simulink model "SimulationLab2"  (R2020a)
settings: Solver=VariableStepAuto  StartTime=0.0  StopTime=20  MaxStep=0.001  RelTol=1e-3
model workspace (MAT data in the model file):
  Phi21 = Simulink.Parameter
  Phi21.DataType = 'auto'
  Phi21.Dimensions = [0 0]
values from neighbouring files (symbols this model uses):
  b = 0.3    [SimLab2_MATLAB.m]
  d0 = 0    [SimLab2_MATLAB.m]
  ddot0 = 0    [SimLab2_MATLAB.m]
  Gamma1 = Gamma(end)    [SimLab2_MATLAB.m]
  Gamma2 = Gamma(1:end-1)    [SimLab2_MATLAB.m]
  H = [0 0 0 1]    [SimLab2_MATLAB.m]
  k = 32    [SimLab2_MATLAB.m]
  K = place(Phi,Gamma,P)    [SimLab2_MATLAB.m]
  L = place(Phi',H',Po)'    [SimLab2_MATLAB.m]
  Lr = place(Phi22',Phi12',Pr)'    [SimLab2_MATLAB.m]
  M = 20    [SimLab2_MATLAB.m]
  m = 1    [SimLab2_MATLAB.m]
  N = Nu + K*Nx    [SimLab2_MATLAB.m]
  noise = 0    [SimLab2_MATLAB.m]
  Phi11 = Phi(end,end)    [SimLab2_MATLAB.m]
  Phi12 = Phi(end,1:end-1)    [SimLab2_MATLAB.m]
  Phi21 = Phi(1:end-1,end)    [SimLab2_MATLAB.m]
  Phi22 = Phi(1:end-1,1:end-1)    [SimLab2_MATLAB.m]
  sat = 10    [SimLab2_MATLAB.m]
  T = 1/f    (= 0.2)    [SimLab2_MATLAB.m]
  xhat0 = 0    [SimLab2_MATLAB.m]
  y0 = 0    [SimLab2_MATLAB.m]
  ydot0 = 0    [SimLab2_MATLAB.m]
undefined symbols (not defined in the file or in its folder): Gamma, Phi
libraries: dspsrcs4 x2
settings Model: Creator=moham  LastModifiedBy=moham

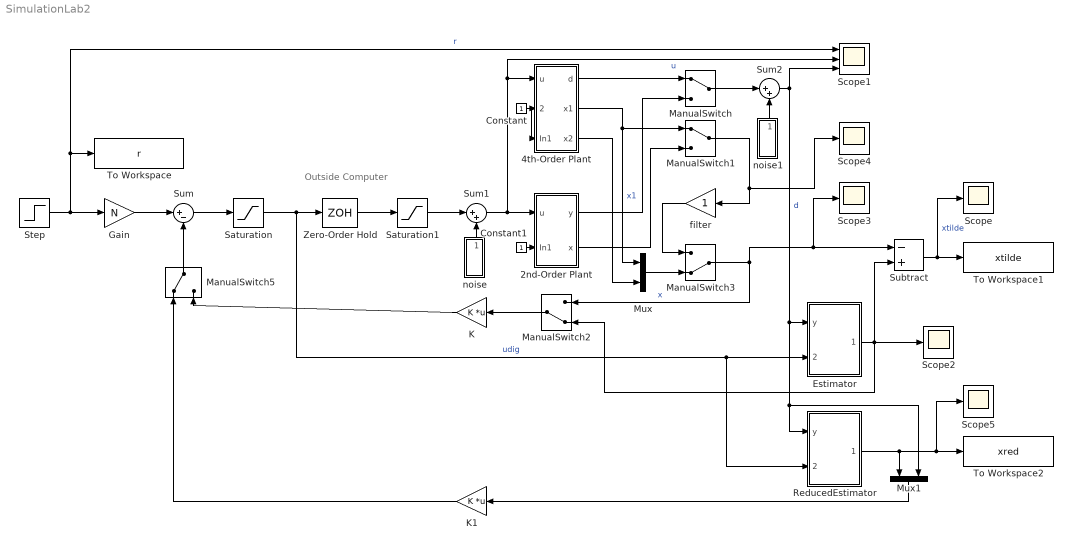
== system SimulationLab2 ==
  note: Outside Computer
  2nd-Order Plant : Subsystem
  4th-Order Plant : Subsystem
  Constant : Constant
  Constant1 : Constant
  Estimator : Subsystem
  Gain : Gain  Gain=N
  K : Gain  Gain=K  Multiplication=Matrix(K*u)
  K1 : Gain  Gain=K  Multiplication=Matrix(K*u)
  ManualSwitch : ManualSwitch
  ManualSwitch1 : ManualSwitch
  ManualSwitch2 : ManualSwitch  CurrentSetting=0
  ManualSwitch3 : ManualSwitch  CurrentSetting=0
  ManualSwitch5 : ManualSwitch
  Mux : Mux  Inputs=2
  Mux1 : Mux  Inputs=2
  ReducedEstimator : Subsystem
  Saturation : Saturate  UpperLimit=sat  LowerLimit=-sat
  Saturation1 : Saturate  UpperLimit=sat  LowerLimit=-sat
  Scope{,2..5} (5 alike) : Scope
  Scope1 : Scope  NumInputPorts=3
  Step : Step  SampleTime=0
  Subtract : Sum  Inputs=-+
  Sum : Sum  Inputs=|+-
  Sum1 : Sum  Inputs=|++
  Sum2 : Sum  Inputs=|++
  To Workspace : ToWorkspace  VariableName=r  SaveFormat=Timeseries  SampleTime=-1
  To Workspace1 : ToWorkspace  VariableName=xtilde  SaveFormat=Timeseries  SampleTime=-1
  To Workspace2 : ToWorkspace  VariableName=xred  SaveFormat=Timeseries  SampleTime=-1
  Zero-Order Hold : ZeroOrderHold  SampleTime=T
  filter : Gain
  noise : Subsystem
      settings: PortSchema="{\"entries\":[{\"content\":{\"sides\":[{\"content\":{\"connectorIds\":[]},\"type\":\"ConnectorPlacement.EquallySpacedRectSide\",\"uuid\":\"5a2ebff0-5337-438e-881a-2a401c8ea54b\"},{\"content\":{\"connectorIds\":[],\"side\":\"RIGHT\"},\"type\":\"ConnectorPlacement.EquallySpacedRectSide\",\"uuid\":\"8a698ae8-d8dc-4938-a16d-c3d33920490f\"},{\"content\":{\"connectorIds\":[\"Out1\"],\"side\":\"TOP\"},\"type\":\"ConnectorPlacement.EquallySpacedRectSide\",\"uuid\":\"6ccd071d-03b7-4ebf-8d4f-7f0039e9795c\"}]},\"type\":\"ConnectorPlacement.EquallySpacedConnector\",\"uuid\":\"f7e7b649-db4e-4589-9059-748e0c795d74\"}],\"packageUris\":[\"http://schema.mathworks.com/mf0/Connector/19700101\"],\"version\":\"1.0\"}"
  noise1 : Subsystem
      settings: PortSchema="{\"entries\":[{\"content\":{\"sides\":[{\"content\":{\"connectorIds\":[]},\"type\":\"ConnectorPlacement.EquallySpacedRectSide\",\"uuid\":\"5a2ebff0-5337-438e-881a-2a401c8ea54b\"},{\"content\":{\"connectorIds\":[],\"side\":\"RIGHT\"},\"type\":\"ConnectorPlacement.EquallySpacedRectSide\",\"uuid\":\"8a698ae8-d8dc-4938-a16d-c3d33920490f\"},{\"content\":{\"connectorIds\":[\"Out1\"],\"side\":\"TOP\"},\"type\":\"ConnectorPlacement.EquallySpacedRectSide\",\"uuid\":\"6ccd071d-03b7-4ebf-8d4f-7f0039e9795c\"}]},\"type\":\"ConnectorPlacement.EquallySpacedConnector\",\"uuid\":\"f7e7b649-db4e-4589-9059-748e0c795d74\"}],\"packageUris\":[\"http://schema.mathworks.com/mf0/Connector/19700101\"],\"version\":\"1.0\"}"
  wires:
  Step/1 -> Scope1/1, To Workspace/1, Gain/1  "r"
  Gain/1 -> Sum/1
  Sum/1 -> Saturation/1
  Saturation/1 -> Zero-Order Hold/1, ReducedEstimator/2(udig), Estimator/2(udig)  "udig"
  Subtract/1 -> To Workspace1/1, Scope/1  "xtilde"
  K/1 -> ManualSwitch5/2
  2nd-Order Plant/1(y) -> ManualSwitch/2
  4th-Order Plant/1(d) -> ManualSwitch/1
  4th-Order Plant/2(x1) -> Mux/1, ManualSwitch1/1  "x1"
  2nd-Order Plant/2(x) -> ManualSwitch1/2
  ManualSwitch/1 -> Sum2/1
  Constant1/1 -> 2nd-Order Plant/2(In1)
  ManualSwitch2/1 -> K/1
  Constant/1 -> 4th-Order Plant/2(dummy), 4th-Order Plant/3(In1)
  4th-Order Plant/3(x2) -> Mux/2
  Mux/1 -> ManualSwitch3/2
  ManualSwitch1/1 -> Scope4/1, filter/1
  filter/1 -> ManualSwitch3/1
  Sum1/1 -> Scope1/2, 4th-Order Plant/1(u), 2nd-Order Plant/1(u)  "u"
  noise/1(noise) -> Sum1/2
  noise1/1(noise) -> Sum2/2
  Sum2/1 -> Scope1/3, Mux1/2, ReducedEstimator/1(y), Estimator/1(y)  "d"
  Zero-Order Hold/1 -> Saturation1/1
  Saturation1/1 -> Sum1/1
  Estimator/1(xhat) -> Subtract/2, Scope2/1, ManualSwitch2/2
  ManualSwitch3/1 -> Scope3/1, Subtract/1, ManualSwitch2/1  "x"
  ReducedEstimator/1(xred) -> To Workspace2/1, Scope5/1, Mux1/1
  Mux1/1 -> K1/1
  K1/1 -> ManualSwitch5/1
  ManualSwitch5/1 -> Sum/2

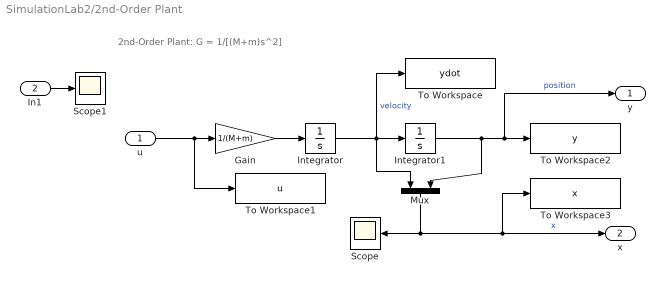
== system SimulationLab2/2nd-Order Plant ==
  note: 2nd-Order Plant: G = 1/[(M+m)s^2]
  u : Inport
  In1 : Inport  Port=2
  Gain : Gain  Gain=1/(M+m)
  Integrator : Integrator
  Integrator1 : Integrator
  Mux : Mux  Inputs=2
  Scope : Scope
  Scope1 : Scope
  To Workspace : ToWorkspace  VariableName=ydot  SaveFormat=Timeseries  SampleTime=-1
  To Workspace1 : ToWorkspace  VariableName=u  SaveFormat=Timeseries  SampleTime=-1
  To Workspace2 : ToWorkspace  VariableName=y  SaveFormat=Timeseries  SampleTime=-1
  To Workspace3 : ToWorkspace  VariableName=x  SaveFormat=Timeseries  SampleTime=-1
  y : Outport  InitialOutput=[0]
  x : Outport  Port=2  InitialOutput=[0]
  wires:
  Gain/1 -> Integrator/1
  u/1 -> Gain/1, To Workspace1/1
  Integrator/1 -> To Workspace/1, Mux/1, Integrator1/1  "velocity"
  Mux/1 -> Scope/1, x/1, To Workspace3/1  "x"
  Integrator1/1 -> y/1, To Workspace2/1, Mux/2  "position"
  In1/1 -> Scope1/1

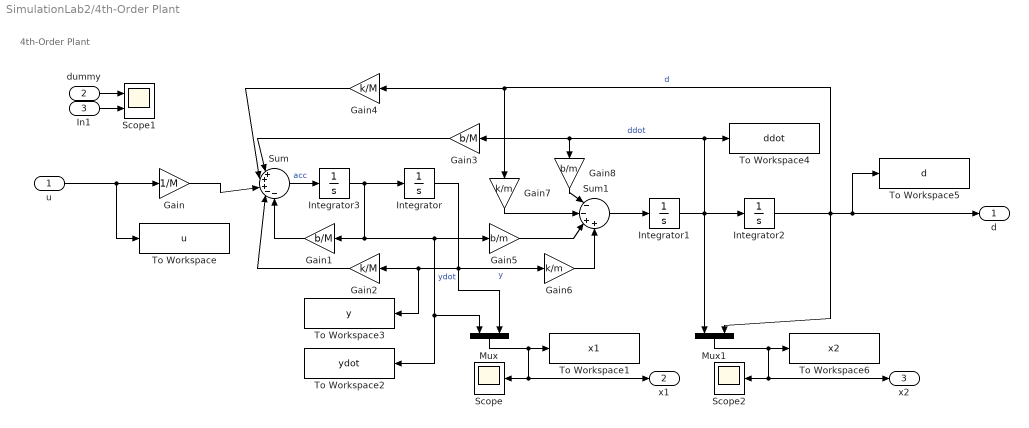
== system SimulationLab2/4th-Order Plant ==
  note: 4th-Order Plant
  u : Inport
  dummy : Inport  Port=2
  In1 : Inport  Port=3
  Gain : Gain  Gain=1/M
  Gain1 : Gain  Gain=b/M
  Gain2 : Gain  Gain=k/M
  Gain3 : Gain  Gain=b/M
  Gain4 : Gain  Gain=k/M
  Gain5 : Gain  Gain=b/m
  Gain6 : Gain  Gain=k/m
  Gain7 : Gain  Gain=k/m
  Gain8 : Gain  Gain=b/m
  Integrator : Integrator  InitialCondition=y0
  Integrator1 : Integrator  InitialCondition=ddot0
  Integrator2 : Integrator  InitialCondition=d0
  Integrator3 : Integrator  InitialCondition=ydot0
  Mux : Mux  Inputs=2
  Mux1 : Mux  Inputs=2
  Scope : Scope
  Scope1 : Scope  NumInputPorts=2
  Scope2 : Scope
  Sum : Sum  Inputs=|+++--
  Sum1 : Sum  Inputs=|--++
  To Workspace : ToWorkspace  VariableName=u  SaveFormat=Timeseries  SampleTime=-1
  To Workspace1 : ToWorkspace  VariableName=x1  SaveFormat=Timeseries  SampleTime=-1
  To Workspace2 : ToWorkspace  VariableName=ydot  SaveFormat=Timeseries  SampleTime=-1
  To Workspace3 : ToWorkspace  VariableName=y  SaveFormat=Timeseries  SampleTime=-1
  To Workspace4 : ToWorkspace  VariableName=ddot  SaveFormat=Timeseries  SampleTime=-1
  To Workspace5 : ToWorkspace  VariableName=d  SaveFormat=Timeseries  SampleTime=-1
  To Workspace6 : ToWorkspace  VariableName=x2  SaveFormat=Timeseries  SampleTime=-1
  d : Outport  InitialOutput=[0]
  x1 : Outport  Port=2  InitialOutput=[0]
  x2 : Outport  Port=3  InitialOutput=[0]
  wires:
  Gain5/1 -> Sum1/3
  Integrator1/1 -> Gain8/1, Gain3/1, To Workspace4/1, Integrator2/1, Mux1/1  "ddot"
  Gain2/1 -> Sum/4
  Integrator2/1 -> Mux1/2, Gain7/1, Gain4/1, d/1, To Workspace5/1  "d"
  Gain4/1 -> Sum/2
  Gain3/1 -> Sum/1
  Mux/1 -> x1/1, Scope/1, To Workspace1/1
  Integrator/1 -> Gain6/1, Mux/2, To Workspace3/1, Gain2/1  "y"
  Gain8/1 -> Sum1/1
  Integrator3/1 -> Integrator/1, Mux/1, To Workspace2/1, Gain5/1, Gain1/1  "ydot"
  Sum/1 -> Integrator3/1  "acc"
  Gain/1 -> Sum/3
  u/1 -> Gain/1, To Workspace/1
  Gain7/1 -> Sum1/2
  Sum1/1 -> Integrator1/1
  Gain1/1 -> Sum/5
  Gain6/1 -> Sum1/4
  dummy/1 -> Scope1/1
  Mux1/1 -> To Workspace6/1, x2/1, Scope2/1
  In1/1 -> Scope1/2

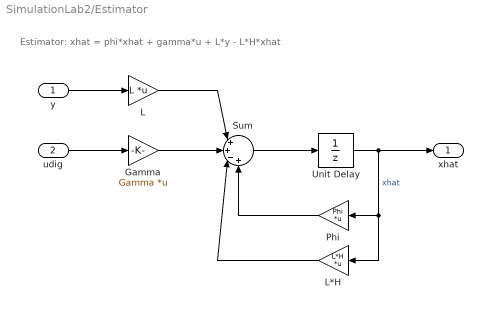
== system SimulationLab2/Estimator ==
  note: Estimator: xhat = phi*xhat + gamma*u + L*y - L*H*xhat
  y : Inport
  udig : Inport  Port=2
  Gamma : Gain  Gain=Gamma  Multiplication=Matrix(K*u)
  L : Gain  Gain=L  Multiplication=Matrix(K*u)
  L*H : Gain  Gain=L*H  Multiplication=Matrix(K*u)
  Phi : Gain  Gain=Phi  Multiplication=Matrix(K*u)
  Sum : Sum  Inputs=|++-+
  Unit Delay : UnitDelay  InitialCondition=xhat0  SampleTime=T  HasFrameUpgradeWarning=on
  xhat : Outport
  wires:
  L*H/1 -> Sum/3
  y/1 -> L/1
  Unit Delay/1 -> xhat/1, L*H/1, Phi/1  "xhat"
  udig/1 -> Gamma/1
  Phi/1 -> Sum/4
  Sum/1 -> Unit Delay/1
  L/1 -> Sum/1
  Gamma/1 -> Sum/2

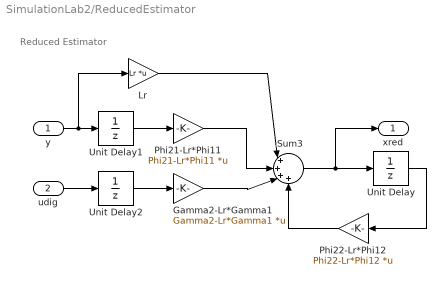
== system SimulationLab2/ReducedEstimator ==
  note: Reduced Estimator
  y : Inport
  udig : Inport  Port=2
  Gamma2-Lr*Gamma1 : Gain  Gain=Gamma2-Lr*Gamma1  Multiplication=Matrix(K*u)
  Lr : Gain  Gain=Lr  Multiplication=Matrix(K*u)
  Phi21-Lr*Phi11 : Gain  Gain=Phi21-Lr*Phi11  Multiplication=Matrix(K*u)
  Phi22-Lr*Phi12 : Gain  Gain=Phi22-Lr*Phi12  Multiplication=Matrix(K*u)
  Sum3 : Sum  Inputs=|++++
  Unit Delay : UnitDelay  SampleTime=T  HasFrameUpgradeWarning=on
  Unit Delay1 : UnitDelay  SampleTime=T  HasFrameUpgradeWarning=on
  Unit Delay2 : UnitDelay  SampleTime=T  HasFrameUpgradeWarning=on
  xred : Outport
  wires:
  Phi21-Lr*Phi11/1 -> Sum3/2
  Phi22-Lr*Phi12/1 -> Sum3/4
  Gamma2-Lr*Gamma1/1 -> Sum3/3
  y/1 -> Lr/1, Unit Delay1/1
  udig/1 -> Unit Delay2/1
  Sum3/1 -> xred/1, Unit Delay/1
  Unit Delay1/1 -> Phi21-Lr*Phi11/1
  Unit Delay2/1 -> Gamma2-Lr*Gamma1/1
  Unit Delay/1 -> Phi22-Lr*Phi12/1
  Lr/1 -> Sum3/1

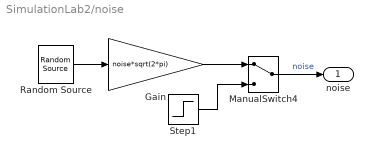
== system SimulationLab2/noise ==
  Gain : Gain  Gain=noise*sqrt(2*pi)
  ManualSwitch4 : ManualSwitch
  Random Source : dspsrcs4/Random Source  SrcType=Gaussian  NormMethod=Ziggurat  CltLength=12  MinVal=0  MaxVal=1  MeanVal=0  VarVal=1  RepMode=Not repeatable  rawSeed=1  IsInherit=off  SampMode=Discrete  SampTime=1e-3  SampFrame=1  DataType=Double  OutComplex=Real  OutputFrames=off
  Step1 : Step  After=noise  SampleTime=0
  noise : Outport
  wires:
  Random Source/1 -> Gain/1
  ManualSwitch4/1 -> noise/1  "noise"
  Step1/1 -> ManualSwitch4/2
  Gain/1 -> ManualSwitch4/1

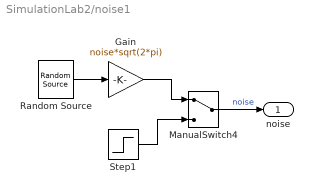
== system SimulationLab2/noise1 ==
  Gain : Gain  Gain=noise*sqrt(2*pi)
  ManualSwitch4 : ManualSwitch
  Random Source : dspsrcs4/Random Source  SrcType=Gaussian  NormMethod=Ziggurat  CltLength=12  MinVal=0  MaxVal=1  MeanVal=0  VarVal=1  RepMode=Not repeatable  rawSeed=1  IsInherit=off  SampMode=Discrete  SampTime=1  SampFrame=1  DataType=Double  OutComplex=Real  OutputFrames=off
  Step1 : Step  After=noise  SampleTime=0
  noise : Outport
  wires:
  Gain/1 -> ManualSwitch4/1
  Step1/1 -> ManualSwitch4/2
  ManualSwitch4/1 -> noise/1  "noise"
  Random Source/1 -> Gain/1
